simulink model "footWater"  (Simulink 7.9)
settings: Solver=ode45  StartTime=0.0  StopTime=10.0  RelTol=1e-3
values from neighbouring files (symbols this model uses):
  water_level = 0    [matlab.mat]    (also in simParam.m; simParams.m; simParams_closed.m; speed_cg.mat)
libraries: mblibv1 x3
settings Model: Creator=nitisht  LastModifiedBy=nitisht
settings ConfigurationSet: Description=SimMechanics 2G

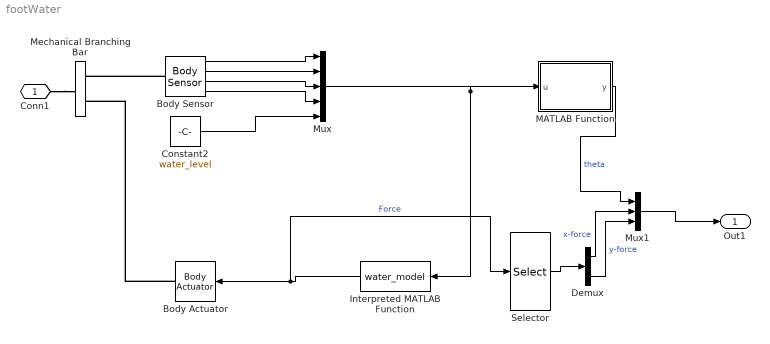
== system footWater ==
  Body Actuator : mblibv1/Sensors &  Actuators/Body Actuator  UpdateFromCAD=off  PhysicalDomain=Mechanical  PortType=blob  ActuationStyle=Force  AngleUnits=deg  ArcVelocityUnits=deg/s  ArcAccelerationUnits=deg/s^2  CoordPositionUnits=m  VelocityUnits=m/s  AccelerationUnits=m/s^2  ForceUnits=N  TorqueUnits=N*m  ActiveIO=off  Width=6  DialogClass=MechanicalActuatorBlock  ReferenceFrame=Absolute (World)  Angle=off  CoordPosition=on  Force=on  Torque=on
  Body Sensor : mblibv1/Sensors &  Actuators/Body Sensor  UpdateFromCAD=off  PhysicalDomain=Mechanical  PortType=blob  Muxed=off  Pose=on  Angle=on  AngleUnits=deg  ArcVelocity=on  ArcVelocityUnits=rad/s  ArcAcceleration=off  ArcAccelerationUnits=deg/s^2  CoordPosition=on  CoordPositionUnits=m  Velocity=on  VelocityUnits=m/s  Acceleration=off  AccelerationUnits=m/s^2  Quaternion=on  QuaternionDT=off  QuaternionDDT=off  QuaternionUnits=off  OutputVector=[1]  ActiveIO=off  Width=18  DialogClass=MechanicalSensorBlock  ReferenceFrame=Absolute (World)
  Constant2 : Constant  Value=water_level
  Demux : Demux  Outputs=2
  Interpreted MATLAB Function : MATLABFcn  MATLABFcn=water_model
  MATLAB Function : MATLAB Function  TreatAsAtomicUnit=on
  Mechanical Branching Bar : mblibv1/Utilities/Mechanical Branching Bar  LConnTagsString=_newl0  RConnTagsString=__newr0|SA2  UpdateFromCAD=off  DialogClass=MechanicalBranchingBarBlock  NumSAPorts=2
  Mux : Mux  Inputs=5
  Mux1 : Mux  Inputs=3
  Selector : Selector  InputPortWidth=6  IndexOptions=Index vector (dialog)  Indices=[4 5]  OutputSizes=1
  Conn1 : PMIOPort  Port=1  Side=Left
  Out1 : Outport
  wires:
  Demux/2 -> Mux1/3  "y-force"
  Demux/1 -> Mux1/2  "x-force"
  Selector/1 -> Demux/1
  Mux1/1 -> Out1/1
  MATLAB Function/1(y) -> Mux1/1  "theta"
  Interpreted MATLAB Function/1 -> Selector/1, Body Actuator/1  "Force"
  Constant2/1 -> Mux/5
  Body Sensor/4 -> Mux/4
  Body Sensor/3 -> Mux/3
  Body Sensor/2 -> Mux/2
  Body Sensor/1 -> Mux/1
  Mux/1 -> MATLAB Function/1(u), Interpreted MATLAB Function/1
  connections:
  Conn1/RConn1 -- Mechanical Branching Bar/LConn1
  Body Sensor/LConn1 -- Mechanical Branching Bar/RConn1
  Body Actuator/RConn1 -- Mechanical Branching Bar/RConn2

== matlab function MATLAB Function ==
  data: u input double; y output double
function y = fcn(u)
%#codegen
    theta = -1*atan2(u(11),u(10));
    
y = theta;
